simulink model "Manipulator_PDControl_InverseDynamics"  (R2020b)
settings: Solver=FixedStepAuto  StartTime=0.0  StopTime=t_final  FixedStep=dt  RelTol=1e-3
values from neighbouring files (symbols this model uses):
  dq_0 = 0.1 *[ 0  -1  0]    [Initialization.m]
  dt = 1.00e-03    (= 0.001)    [Initialization.m]
  ikInitGuessSim = ikInitGuess    [generateTrajectory.m]
  q_0 = [0;-0.9;2.7]    [Initialization.m]
  waypointAccels = zeros(size(waypointVels))    [generateTrajectory.m]
  waypoints = initPosition +              [0 0 0 ; 0 -a -a ; 0 0 -2*a; 0 a -a ; 0 0 0]'    [generateTrajectory.m]
  waypointVels = 0.1 *[ 0  -1  0 ... (first row only)    [generateTrajectory.m]
libraries: robotcorelib x2, simulink x2, robotmaniplib x1
settings Model: Creator=m2aali  LastModifiedBy=Kons
settings DataIOCC: LoggingToFile=on

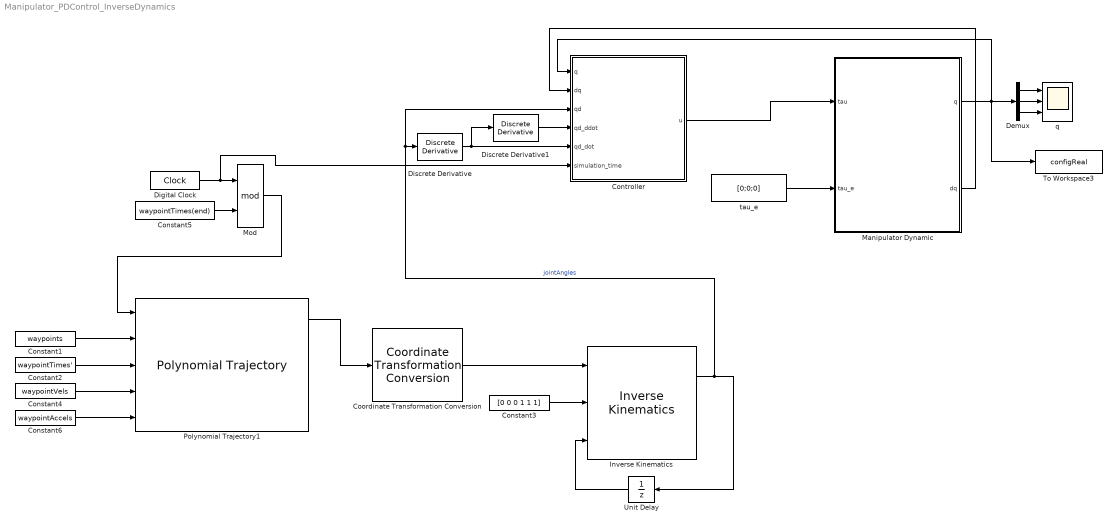
== system Manipulator_PDControl_InverseDynamics ==
  Constant1 : Constant  Value=waypoints  VectorParams1D=off  SampleTime=-1
  Constant2 : Constant  Value=waypointTimes'  VectorParams1D=off  SampleTime=-1
  Constant3 : Constant  Value=[0 0 0 1 1 1]  VectorParams1D=off
  Constant4 : Constant  Value=waypointVels  VectorParams1D=off  SampleTime=-1
  Constant5 : Constant  Value=waypointTimes(end)
  Constant6 : Constant  Value=waypointAccels  VectorParams1D=off  SampleTime=-1
  Controller : Subsystem
  Coordinate Transformation Conversion : robotcorelib/Coordinate Transformation Conversion  InputRepresentation=Translation Vector  InputEulerSequence=ZYX  ShowTrVecInputPort=on  OutputRepresentation=Homogeneous Transformation  OutputEulerSequence=ZYX  ShowTrVecOutputPort=on  SimulateUsing=Code generation
      settings: SourceProductBaseCode=NV,RO,RR,UV
  Demux : Demux  Outputs=3
  Digital Clock : DigitalClock  SampleTime=dt
  Discrete Derivative : simulink/Discrete/Discrete Derivative  gainval=1.0  ICPrevScaledInput=[-0.000001274337461;-0.900000000000479;2.699999999999876]*1000  OutMin=[]  OutMax=[]  OutDataType=fixdt(1, 16)  OutScaling=2^-10  DoSatur=off
  Discrete Derivative1 : simulink/Discrete/Discrete Derivative  gainval=1.0  ICPrevScaledInput="[ 0 ; 0;  0]"  OutMin=[]  OutMax=[]  OutDataType=fixdt(1, 16)  OutScaling=2^-10  DoSatur=off
  Inverse Kinematics : robotmaniplib/Inverse Kinematics  RigidBodyTree=robot  EndEffector=Link_EE  ShowInfo=on  SolverName=BFGS Gradient Projection  EnforceJointLimits=on  MaxIterations=1500  MaxTime=10  GradientTolerance=1e-7  SolutionTolerance=1e-6  StepTolerance=1e-14  ErrorChangeTolerance=1e-12  UseErrorDamping=on  DampingBias=0.0025  SimulateUsing=Code generation
  Manipulator Dynamic : Subsystem
  Mod : Math  Operator=mod  SignedPower=on  SaturateOnIntegerOverflow=on
  Polynomial Trajectory1 : robotcorelib/Polynomial Trajectory  WaypointSource=External  Waypoints=[ 0, 2, 1, 5, 0; -1, 3, 1, 4, 4 ]  TimePoints=[ 0, 1, 2, 3, 4 ]  TimeInterval=[ 1, 4 ]  Method=Quintic Polynomial  ParameterSource=External  VelocityBoundaryCondition=zeros( 2, 5 )  AccelerationBoundaryCondition=zeros( 2, 5 )  SimulateUsing=Code generation
  To Workspace3 : ToWorkspace  VariableName=configReal  SaveFormat=Timeseries  SampleTime=-1
  Unit Delay : UnitDelay  InitialCondition=ikInitGuessSim  SampleTime=-1  HasFrameUpgradeWarning=on
  q : Scope  NumInputPorts=3
  tau_e : Constant  Value=[0;0;0]
  wires:
  tau_e/1 -> Manipulator Dynamic/2(tau_e)
  Manipulator Dynamic/2(dq) -> Controller/2(dq)
  Controller/1(u) -> Manipulator Dynamic/1(tau)
  Demux/1 -> q/1
  Demux/2 -> q/2
  Demux/3 -> q/3
  Digital Clock/1 -> Controller/6(simulation_time), Mod/1
  Mod/1 -> Polynomial Trajectory1/1
  Constant5/1 -> Mod/2
  Polynomial Trajectory1/1 -> Coordinate Transformation Conversion/1
  Inverse Kinematics/1 -> Unit Delay/1, Controller/3(qd), Discrete Derivative/1  "jointAngles"
  Unit Delay/1 -> Inverse Kinematics/3
  Constant3/1 -> Inverse Kinematics/2
  Coordinate Transformation Conversion/1 -> Inverse Kinematics/1
  Discrete Derivative1/1 -> Controller/4(qd_ddot)
  Discrete Derivative/1 -> Discrete Derivative1/1, Controller/5(qd_dot)
  Constant1/1 -> Polynomial Trajectory1/2
  Constant2/1 -> Polynomial Trajectory1/3
  Constant4/1 -> Polynomial Trajectory1/4
  Constant6/1 -> Polynomial Trajectory1/5
  Manipulator Dynamic/1(q) -> To Workspace3/1, Demux/1, Controller/1(q)

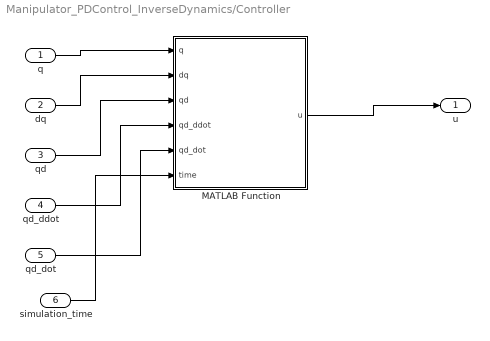
== system Manipulator_PDControl_InverseDynamics/Controller ==
  q : Inport
  dq : Inport  Port=2
  qd : Inport  Port=3
  qd_ddot : Inport  Port=4
  qd_dot : Inport  Port=5
  simulation_time : Inport  Port=6
  MATLAB Function : MATLAB Function  TreatAsAtomicUnit=on
  u : Outport
  wires:
  dq/1 -> MATLAB Function/2(dq)
  MATLAB Function/1(u) -> u/1
  qd/1 -> MATLAB Function/3(qd)
  q/1 -> MATLAB Function/1(q)
  qd_ddot/1 -> MATLAB Function/4(qd_ddot)
  qd_dot/1 -> MATLAB Function/5(qd_dot)
  simulation_time/1 -> MATLAB Function/6(time)

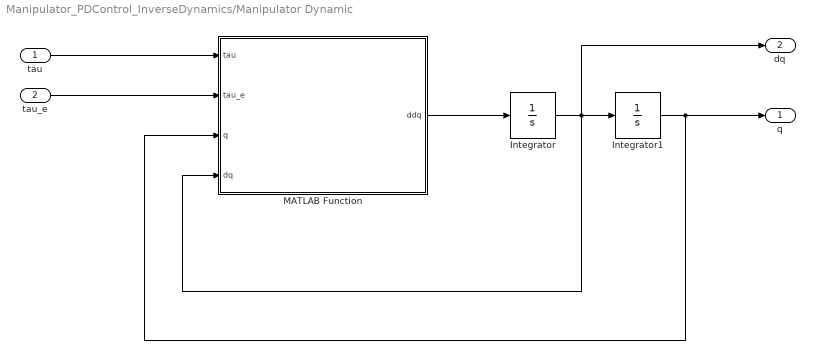
== system Manipulator_PDControl_InverseDynamics/Manipulator Dynamic ==
  tau : Inport
  tau_e : Inport  Port=2
  Integrator : Integrator  InitialCondition=dq_0
  Integrator1 : Integrator  InitialCondition=q_0
  MATLAB Function : MATLAB Function  TreatAsAtomicUnit=on
  q : Outport
  dq : Outport  Port=2
  wires:
  MATLAB Function/1(ddq) -> Integrator/1
  tau/1 -> MATLAB Function/1(tau)
  tau_e/1 -> MATLAB Function/2(tau_e)
  Integrator1/1 -> q/1, MATLAB Function/3(q)
  Integrator/1 -> dq/1, MATLAB Function/4(dq), Integrator1/1

== matlab function Manipulator_PDControl_InverseDynamics/Controller/MATLAB Function ==
  data: q input; dq input; u output; qd input; qd_ddot input; qd_dot input; time input
function u = fcn(q, dq, qd,  qd_ddot, qd_dot, time)
% PD + gravity compensation controller function

%% reset first qd_ddot
if (time < 0.003)
    qd_ddot = [0;0;0];
    qd_dot = [0;0;0];
end
%% general physical parameters

l1 = 0.6731;
l2 = 0.432;
l3 = 0.434;
lc2 = 0.216;
lc3 = 0.164;
m2 = 15.46;
m3 = 9.55;
J = 0.302;


%% Joint Space variables

q1 = q(1);
q2 = q(2);
q3 = q(3);

dq1 = dq(1);
dq2 = dq(2);
dq3 = dq(3);
g = 9.81;

%% Inertia Matrix Parameters

J1 = m3 * lc3^2;
J12 = (m2 * lc2^2) + (m3 * l2^2);
J13 = l2 * lc3 * m3;


h11 = J + J1 * (sin(q2 + q3))^2 + J12 * (cos(q2))^2 + 2 * J13 * cos(q2) * sin(q2+q3);
h22 = J1 + J12 + 2 * J13 * sin(q3);
h23 = J1 + J13 * sin(q3);
h32 = h23;
h33 = J1;

H = [h11, 0 ,0 ;
    0 , h22, h23;
    0 , h32, h33];

%% Matrix C defining the Coriolis and centrifugal generalized forces

c12_1 = J1 * sin(2 * (q1 + q2)) - J12 * sin(2 * q2) + 2 * J13 * cos(2 * q2 +q3);
c13_1 = J1 * sin(2 * (q2 + q3)) + 2 * J13 * cos(q2) * cos(q2 + q3);
c11_2 = (1/2) * (-J1 * sin(2 * (q2 + q3)) + J12 * sin(2 * q2) - 2 * J13 * cos(2 * q2 + q3));
c22_2 = 2 * J13 * cos(q3);
c23_2 = J13 * cos(q3);
c22_3 = -J13 * cos(q3) * dq2;
c11_3 = (-1/2) * (J1 * sin(2 * (q2 + q3)) + J13 * cos(q2) * cos(q2 + q3));

C = [0, c12_1 * dq1, c13_1 * dq3;
    c11_2 * dq1, 0 , c22_2 * dq2 + c23_2 * dq3;
    c11_3 * dq1, c22_3 * dq2, 0];


%% Vector of Potential Forces Parameters

g21 = -g * (lc3 * m3 * sin(q2 + q3) + lc2 * m2 * cos(q2) + l2 * m3 * cos(q2));
g31 = -g * (lc3 * m3 * sin(q2 + q3));

G = [0;
    g21;
    g31];

%% PD Controller Parameters 

Kp = [20,0,0; 0, 10 ,0; 0, 0 , 10];  %  Kp is 3*3 matrix of proportional gain 
Kd = [1,0,0; 0, 1 ,0; 0, 0 , 1]; %Kd is 3*3 matrix of derivative gain

%% Control Law

aq = qd_ddot - Kp * (q - qd) - Kd * (dq - qd_dot);

%% Control law

u = H * aq + C * dq + G;
% u = - Kp * (q - qd) - Kd * dq + G;

== matlab function Manipulator_PDControl_InverseDynamics/Manipulator Dynamic/MATLAB Function ==
  data: tau input; tau_e input; q input; ddq output; dq input
function ddq = DynamicModel( tau, tau_e, q, dq)
%%%%%
% 3-DOF Puma-560 Dynamic Model Function
% H(q)* ddq + C(q) * dq + G = tau + tau_e
% q is 3*1 vector of joint variables (radian)
% H(q) is the inertia matrix
% C(q) is the matrix of Coriolis and centrifugal forces
% G(q) is  the vector of potential forces Parameters
% tau is control torque 
% tau_e is the external torque due to the interaction with the environment
%%%%%

%% Joint Space variables

q1 = q(1);
q2 = q(2);
q3 = q(3);

dq1 = dq(1);
dq2 = dq(2);
dq3 = dq(3);

%% general physical parameters

l1 = 0.6731;
l2 = 0.432;
l3 = 0.434;
lc2 = 0.216;
lc3 = 0.164;
m2 = 15.46;
m3 = 9.55;
J = 0.302;

%% Inertia Matrix Parameters

J1 = m3 * lc3^2;
J12 = (m2 * lc2^2) + (m3 * l2^2);
J13 = l2 * lc3 * m3;


h11 = J + J1 * (sin(q2 + q3))^2 + J12 * (cos(q2))^2 + 2 * J13 * cos(q2) * sin(q2+q3);
h22 = J1 + J12 + 2 * J13 * sin(q3);
h23 = J1 + J13 * sin(q3);
h32 = h23;
h33 = J1;

H = [h11, 0 ,0 ;
    0 , h22, h23;
    0 , h32, h33];

%% Coriolis Matrix Parameters

c12_1 = J1 * sin(2 * (q1 + q2)) - J12 * sin(2 * q2) + 2 * J13 * cos(2 * q2 +q3);
c13_1 = J1 * sin(2 * (q2 + q3)) + 2 * J13 * cos(q2) * cos(q2 + q3);
c11_2 = (1/2) * (-J1 * sin(2 * (q2 + q3)) + J12 * sin(2 * q2) - 2 * J13 * cos(2 * q2 + q3));
c22_2 = 2 * J13 * cos(q3);
c23_2 = J13 * cos(q3);
c22_3 = -J13 * cos(q3) * dq2;
c11_3 = (-1/2) * (J1 * sin(2 * (q2 + q3)) + J13 * cos(q2) * cos(q2 + q3));

C = [0, c12_1 * dq1, c13_1 * dq3;
    c11_2 * dq1, 0 , c22_2 * dq2 + c23_2 * dq3;
    c11_3 * dq1, c22_3 * dq2, 0];

%% Vector of Potential Forces Parameters

g = 9.81;

g21 = -g * (lc3 * m3 * sin(q2 + q3) + lc2 * m2 * cos(q2) + l2 * m3 * cos(q2));
g31 = -g * (lc3 * m3 * sin(q2 + q3));

G = [0;
    g21;
    g31];

%% Function output

ddq = inv(H)*(tau + tau_e - C * dq - G);
